simulink subsystem "HFUC_8_2A"  (R2024a)
settings: Solver=VariableStepAuto  StartTime=0.0  StopTime=10.0  RelTol=1e-3
libraries: fl_lib x17, sdl_lib x2
settings Model: DefaultTestHarness=HFUC_8_2A_Harness1  Creator=upattacini  LastModifiedBy=upattacini

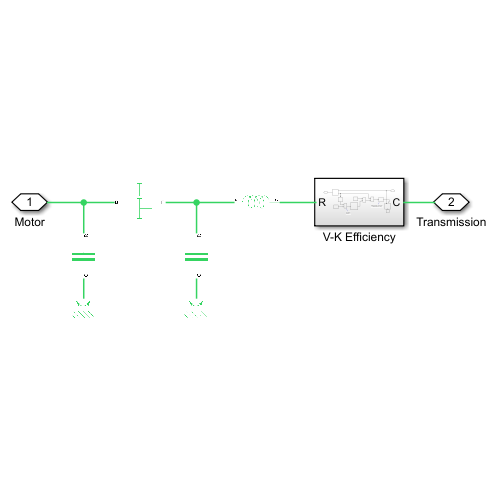
[thumbnail: Simulink's stored preview of the top-level diagram]
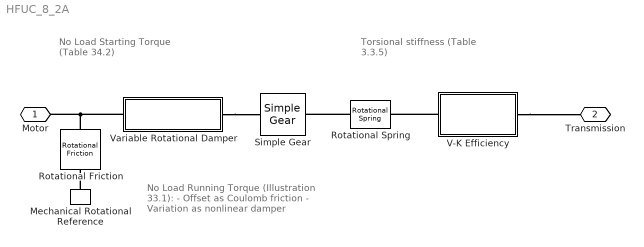
== system HFUC_8_2A ==
  note: Torsional stiffness
      | (Table 3.3.5)
  note: No Load Running Torque (Illustration 33.1):
      | - Offset as Coulomb friction
      | - Variation as nonlinear damper
  note: No Load Starting Torque
      | (Table 34.2)
  Mechanical Rotational Reference : fl_lib/Mechanical/Rotational Elements/Mechanical Rotational Reference
  Rotational Friction : fl_lib/Mechanical/Rotational Elements/Rotational Friction  brkwy_trq=0.59 N*cm  brkwy_vel=0.01 rad/s  Col_trq=0.3 N*cm  visc_coef=0 N*cm*s/rad  w_specify=off  w_priority=None  w=0 rad/s  w_nominal_specify=off  w_nominal_value=1  w_nominal_unit=rad/s  t_specify=off  t_priority=None  t=0 N*m  t_nominal_specify=off  t_nominal_value=1  t_nominal_unit=N*m
  Rotational Spring : fl_lib/Mechanical/Rotational Elements/Rotational Spring  spr_rate=1000 N*m/rad  w_specify=off  w_priority=None  w=0 rad/s  w_nominal_specify=off  w_nominal_value=1  w_nominal_unit=rad/s  t_specify=off  t_priority=None  t=0 N*m  t_nominal_specify=off  t_nominal_value=1  t_nominal_unit=N*m  phi_specify=off  phi_priority=High  phi=0 rad  phi_nominal_specify=off  phi_nominal_value=1  phi_nominal_unit=rad
  Simple Gear : sdl_lib/Gears/Simple Gear  ratio=100  rotation_direction=sdl.enum.shaftOutputDirection.opposite  enable_faults=simscape.enum.onoff.off  efficiency_fault=0.05  fault_angles=pi / 12 rad  friction_model=sdl.enum.gear_efficiencies_load.constant  T_noload=0.1 N*m  T_nom=5 N*m  efficiency_nom=0.8  efficiency=0.8/0.9  temperature_TLU=[280, 300, 320] K  load_TLU=[1, 5, 10] N*m  efficiency_TLU=[.95, .9, .85]  efficiency_TLU2=[.85, .8, .75; .95, .9, .85; .85, .8, .7]  w_thr=0.01 rad/s  pwr_thr=0.001 W  enable_backlash=false  hardstop_model=simscape.enum.hardstop.smooth  backlash_distance=1e-3 mm  r_base=0.1 m  transition=1e-4 mm  backlash_stiffness=1e6 N/m  backlash_damping=1e3 N*s/m  coeff_rest=0.7  v_tol=0.001 m/s  f_tol=0.001 N  mu_visc=[0, 0] N*cm*s/rad  thermal_mass=50 J/K  temperature_specify=off  temperature_priority=High  temperature=300 K  temperature_nominal_specify=off  temperature_nominal_value=1  temperature_nominal_unit=K  x_backlash_specify=off  x_backlash_priority=None  x_backlash=0 mm  x_backlash_nominal_specify=off  x_backlash_nominal_value=1  x_backlash_nominal_unit=mm  f_hardstop_specify=off  f_hardstop_priority=None  f_hardstop=0 N  f_hardstop_nominal_specify=off  f_hardstop_nominal_value=1  f_hardstop_nominal_unit=N  v_backlash_specify=off  v_backlash_priority=None  v_backlash=0 m/s  v_backlash_nominal_specify=off  v_backlash_nominal_value=1  v_backlash_nominal_unit=m/s
  V-K Efficiency : Subsystem
  Variable Rotational Damper : Subsystem
      mask Display: disp('Variable Rotational\nDamper');
  Motor : PMIOPort  Side=Left
  Transmission : PMIOPort  Port=2  Side=Right
  connections:
  Variable Rotational Damper/LConn1 -- Rotational Friction/LConn1 -- Motor/RConn1
  V-K Efficiency/LConn1 -- Rotational Spring/RConn1
  V-K Efficiency/RConn1 -- Transmission/RConn1
  Mechanical Rotational Reference/LConn1 -- Rotational Friction/RConn1
  Rotational Spring/LConn1 -- Simple Gear/RConn1
  Variable Rotational Damper/RConn1 -- Simple Gear/LConn1

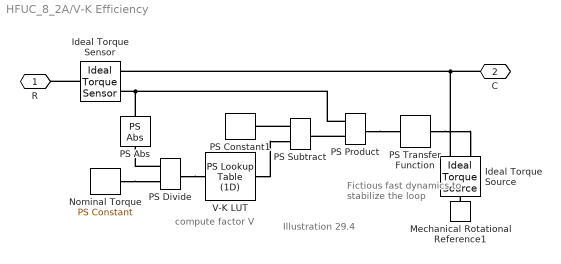
== system HFUC_8_2A/V-K Efficiency ==
  note: compute
      | factor V
  note: Fictious fast dynamics
      | to stabilize the loop
  note: Illustration 29.4
  Ideal Torque Sensor : fl_lib/Mechanical/Mechanical Sensors/Ideal Torque Sensor
  Ideal Torque Source : fl_lib/Mechanical/Mechanical Sources/Ideal Torque Source
  Mechanical Rotational Reference1 : fl_lib/Mechanical/Rotational Elements/Mechanical Rotational Reference
  Nominal Torque : fl_lib/Physical Signals/Sources/PS Constant  constant=2.4 N*m
  PS Abs : fl_lib/Physical Signals/Nonlinear Operators/PS Abs
      settings: InternalSimscapePortConfiguration="{\"Bottom\":[],\"Left\":[{\"id\":\"I\",\"label\":\"\",\"type\":\"input\"}],\"Right\":[{\"id\":\"O\",\"label\":\"\",\"type\":\"output\"}],\"Top\":[]}"
  PS Constant1 : fl_lib/Physical Signals/Sources/PS Constant  constant=1
  PS Divide : fl_lib/Physical Signals/Functions/PS Divide
  PS Product : fl_lib/Physical Signals/Functions/PS Product
  PS Subtract : fl_lib/Physical Signals/Functions/PS Subtract
  PS Transfer Function : fl_lib/Physical Signals/Linear Operators/PS Transfer Function  transfer_function_type=foundation.enum.transfer_function_type.lag  T=1e-6 s  T1=2 s  T2=1 s  reset_method=foundation.enum.IntegratorResetSpec.None  initial_condition_spec=foundation.enum.IntegratorICSpec.Internal  y0=0 N*m
      settings: InternalSimscapePortConfiguration="{\"Bottom\":[],\"Left\":[{\"id\":\"U\",\"label\":\"\",\"type\":\"input\"}],\"Right\":[{\"id\":\"Y\",\"label\":\"\",\"type\":\"output\"}],\"Top\":[]}"
  V-K LUT : fl_lib/Physical Signals/Lookup Tables/PS Lookup Table (1D)  x=[0.1, 0.2, 0.4, 0.6, 0.8, 1]  f=[0.45, 0.65, 0.85, 0.95, 0.99, 1]  interp_method=simscape.enum.interpolation.linear  extrap_method=simscape.enum.extrapolation.nearest
  R : PMIOPort  Side=Left
  C : PMIOPort  Port=2  Side=Right
  connections:
  PS Divide/LConn1 -- PS Abs/RConn1
  PS Abs/LConn1 -- PS Product/LConn1 -- Ideal Torque Sensor/RConn2
  Ideal Torque Sensor/LConn1 -- R/RConn1
  C/RConn1 -- Ideal Torque Source/RConn2 -- Ideal Torque Sensor/RConn1
  Nominal Torque/RConn1 -- PS Divide/LConn2
  PS Divide/RConn1 -- V-K LUT/LConn1
  PS Subtract/LConn1 -- PS Constant1/RConn1
  V-K LUT/RConn1 -- PS Subtract/LConn2
  PS Product/LConn2 -- PS Subtract/RConn1
  PS Product/RConn1 -- PS Transfer Function/LConn1
  Mechanical Rotational Reference1/LConn1 -- Ideal Torque Source/LConn1
  PS Transfer Function/RConn1 -- Ideal Torque Source/RConn1

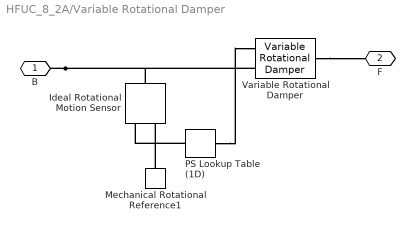
== system HFUC_8_2A/Variable Rotational Damper ==
  Ideal Rotational Motion Sensor : fl_lib/Mechanical/Mechanical Sensors/Ideal Rotational Motion Sensor  reference=foundation.enum.MeasurementReference.difference  acceleration_port=false  velocity_port=true  position_port=false  wrap_angle=false  offset=0 rad
      settings: InternalSimscapePortConfiguration="{\"Bottom\":[],\"Left\":[{\"id\":\"R\",\"label\":\"R\",\"type\":\"foundation.mechanical.rotational.rotational\"}],\"Right\":[{\"id\":\"C\",\"label\":\"C\",\"type\":\"foundation.mechanical.rotational.rotational\"},{\"id\":\"W\",\"label\":\"W\",\"type\":\"output\"}],\"Top\":[]}"
  Mechanical Rotational Reference1 : fl_lib/Mechanical/Rotational Elements/Mechanical Rotational Reference
  PS Lookup Table (1D) : fl_lib/Physical Signals/Lookup Tables/PS Lookup Table (1D)  x=[500, 1000, 2000, 3500] rpm  f=[0, 0.1, 0.2, 0.7] N*cm/rpm  interp_method=simscape.enum.interpolation.linear  extrap_method=simscape.enum.extrapolation.nearest
  Variable Rotational Damper : sdl_lib/Couplings & Drives/Springs & Dampers/Variable Rotational Damper  Bmin=0.01 N*cm/rpm
      settings: InternalSimscapePortConfiguration="{\"Bottom\":[],\"Left\":[{\"id\":\"B\",\"label\":\"B\",\"type\":\"input\"},{\"id\":\"R\",\"label\":\"R\",\"type\":\"foundation.mechanical.rotational.rotational\"}],\"Right\":[{\"id\":\"C\",\"label\":\"C\",\"type\":\"foundation.mechanical.rotational.rotational\"}],\"Top\":[]}"
  B : PMIOPort  Side=Left
  F : PMIOPort  Port=2  Side=Right
  connections:
  PS Lookup Table (1D)/RConn1 -- Variable Rotational Damper/LConn1
  Variable Rotational Damper/RConn1 -- F/RConn1
  B/RConn1 -- Variable Rotational Damper/LConn2 -- Ideal Rotational Motion Sensor/LConn1
  PS Lookup Table (1D)/LConn1 -- Ideal Rotational Motion Sensor/RConn2
  Mechanical Rotational Reference1/LConn1 -- Ideal Rotational Motion Sensor/RConn1
